simulink model "ForceReadingTCP"  (R2025b)
settings: Solver=VariableStepAuto  StartTime=0.0  StopTime=25  RelTol=1e-3
undefined symbols (not defined in the file or in its folder): f
libraries: instrumentlib x1
settings Model: Creator=mmm_r  LastModifiedBy=mmm_r

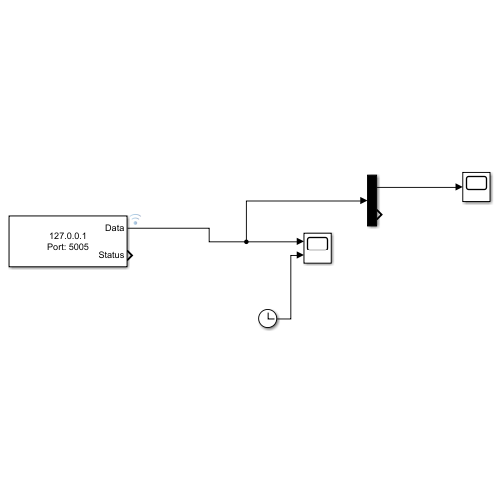
[thumbnail: Simulink's stored preview of the top-level diagram]
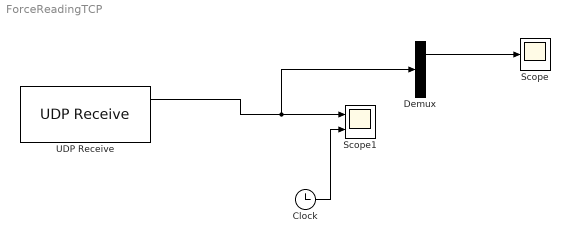
== system ForceReadingTCP ==
  Clock : Clock
  Demux : Demux  Outputs=2
  Scope : Scope
      settings: ActiveDisplayYMinimum=0.53047397410550068  ActiveDisplayYMaximum=2.0300958712776174
  Scope1 : Scope  NumInputPorts=2
      settings: ActiveDisplayYMinimum=-0.95706686930091145  ActiveDisplayYMaximum=5.2701367781155017
  UDP Receive : instrumentlib/UDP Receive  LocalAddress=127.0.0.1  LocalPort=5005  EnablePortSharing=off  Host=0.0.0.0  Port=9090  GetLatestData=on  DataSize=[ 1, 2 ]  DataType=double  ASCIIFormatting=%f,  Terminator=LF  CustomTerminator=10  ByteOrder=little-endian  EnableBlockingMode=off  Timeout=10  SampleTime=0.05  SimulateUsing=Interpreted execution
  wires:
  UDP Receive/1 -> Demux/1, Scope1/1
  Clock/1 -> Scope1/2
  Demux/1 -> Scope/1
